simulink library "cstblocks"  (R2025b)
settings: Solver=ode45  StartTime=0.0  StopTime=10.0  RelTol=1e-3
values from neighbouring files (symbols this model uses):
  D = ltipack.lftdataFRD(IC,ltipack.LFTBlockWrapper(blk))    [ControlDesignBlock.m]    (also in DynamicBlock.m = pidstd(ltipack_ssdata(blk)); delayss.m = ltipack.ssdata(a0,b,c,[d0 q;s zeros(length(tau))],[],Ts))
  Ts = blk.Ts_    [DynamicBlock.m]    (also in delayss.m = varargin{1})
undefined symbols (not defined in the file or in its folder): AA, BB, CC, DD, Discrete, INFO, rss, set, Time, uDelay, V, xinit, yDelay
libraries: $bdroot x4, slpidlib x4, cstextras x4, sharedTrackingLibrary x3, ctrlSharedLib x1
(part 1 of 3)
settings Model: RequirementInfo=9  FPTRunName=Active  Creator=The MathWorks, Inc.  LastModifiedBy=The MathWorks, Inc.
settings SolverCC: AlgebraicLoopSolver=TrustRegion  MaxZcPerStep=1.0
settings DataIOCC: LimitDataPoints=on  SaveFormat=Array  SignalLoggingSaveFormat=ModelDataLogs  ReturnWorkspaceOutputs=off
settings OptimizationCC: BlockReduction=off  BooleanDataType=off  ExpressionDepthLimit=2147483647.0  LifeSpan=inf
settings DebuggingCC: SaveWithParameterizedLinksMsg=none  UnderspecifiedInitializationDetection=Classic  MergeDetectMultiDrivingBlocksExec=none  SignalResolutionControl=TryResolveAllWithWarning  FcnCallInpInsideContextMsg=warning  UnconnectedInputMsg=warning  UnconnectedOutputMsg=warning  UnconnectedLineMsg=warning  StateNameClashWarn=warning  SFUnexpectedBacktrackingDiag=warning  SFNoUnconditionalDefaultTransitionDiag=warning  SFExecutionAtInitializationDiag=none  ArithmeticOperatorsInVariantConditions=warning
settings HardwareCC: ProdBitPerPointer=32.0  ProdBitPerSizeT=32.0  ProdBitPerPtrDiffT=32.0  ProdLargestAtomicFloat=None  ProdIntDivRoundTo=Undefined  ProdEndianess=Unspecified  ProdWordSize=32.0  ProdHWDeviceType=32-bit Generic  TargetUnknown=on
settings ModelReferenceCC: EnableRefExpFcnMdlSchedulingChecks=on  PropagateSignalLabelsOutOfModel=off
settings SFSimCC: SimUseLocalCustomCode=off  CustomCodeUndefinedFunction=UseInterfaceOnly
settings RTWCC: RTWUseLocalCustomCode=off  GPUComputeCapability=3.5  DLArmComputeVersion=19.05  LargeConstantGeneration=WriteOnlyDNNConstantsToDataFiles
settings CodeAppCC: StateflowObjectComments=on
settings GRTTargetCC: TargetLangStandard=C89/C90 (ANSI)  CombineOutputUpdateFcns=off  GRTInterface=on
settings ConfigComp: CovMetricSettings=dw  CovSaveCumulativeToWorkspaceVar=on  CovSaveSingleToWorkspaceVar=on  CovExternalEMLEnable=off  CovSFcnEnable=off

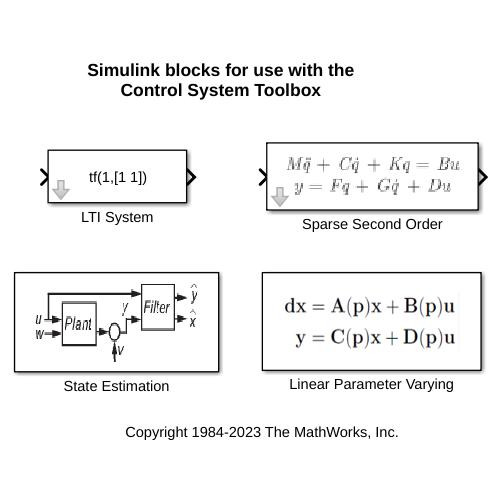
[thumbnail: Simulink's stored preview of the top-level diagram]
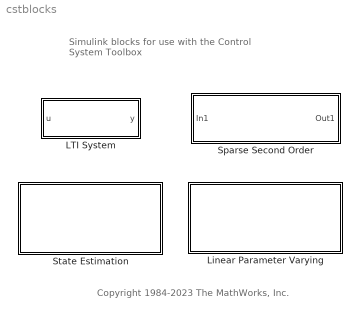
== system cstblocks ==
  note: Simulink blocks for use with the
      | Control System Toolbox
  note: Copyright 1984-2023 The MathWorks, Inc.
  LTI System : Subsystem  BlockChoice=CSS  mask(LTI Block){sys=tf(1,[1 1]), IC=[], PadeOrder=0}
      mask prompts: sys "Control:simulink:LTIMaskLabel1"; IC "Control:simulink:LTIMaskLabel2"; PadeOrder "Pade Order (for linearization)"
      mask help: Control:simulink:LTIMaskDescription
      mask init:
      | model = bdroot;
      | df = get_param(model,'dirty');
      | try
      |     [D,uDelay,yDelay,xinit,Ts,sysname] = controllib.internal.blocks.lti.ltimaskData(gcb,sys,IC);
      | catch ME
      |     sysname = '???';
      |     throwAsCaller(MSLException(get_param(gcb,'handle'),ME.identifier,ME.message))
      | end
      | controllib.internal.blocks.lti.ltimaskUpdate(gcb,D,xinit,Ts,PadeOrder)
      | try
      |     % Attempt to modify locked library -> error
      |     set_param(model,'dirty',df)
      | end
      mask Help: eval('helpview(''control'',''ltisystemblock'');')
      mask Callback sys: controllib.internal.blocks.lti.ltimaskCallback(gcb,'System')
      mask DialogControl sys Prompt: LTI system variable
      mask DialogControl IC Prompt: Initial states (state-space only)
      mask Display: disp(sysname)
  Linear Parameter Varying : Subsystem
      mask Display: image('lpv.png',[.1 .2 .8 .6])
  Sparse Second Order : Subsystem  mask(Sparse Second Order){M=1, C=0, K=1, B=1, F=1, G=0, D=0, q0=0, dq0=0}
      mask prompts: M "Control:simulink:SparseSecondOrder1"; C "Control:simulink:SparseSecondOrder2"; K "Control:simulink:SparseSecondOrder3"; q0 "Control:simulink:SparseSecondOrder4"; dq0 "Control:simulink:SparseSecondOrder5"
      mask help: Control:simulink:SSODescription
      mask init:
      | hCB = get_param(gcb,'handle');  % block handle
      | try
      |    sys = mechss(M,C,K,B,F,G,D);
      |    [AA,BB,CC,DD,EE] = sparssdata(sys);
      |    x0 = getx0(sys,q0,dq0);
      | catch ME
      |    throwAsCaller(MSLException(hCB, ME.identifier, ME.message));
      | end
      mask Help: eval('helpview(''control'',''ssoblock'');')
      mask DialogControl M Prompt: M (mass):
      mask DialogControl C Prompt: C (damping):
      mask DialogControl K Prompt: K (stiffness):
      mask DialogControl q0 Prompt: Initial position q(0):
      mask DialogControl dq0 Prompt: Initial velocity q'(0):
  State Estimation : Subsystem
      mask Display: image('kalman.png',[0.1 0.1 0.8 0.8])

== system cstblocks/LTI System ==
  u : Inport  PortDimensions=1  SampleTime=Ts
  Input Delay : $bdroot/Linear Parameter Varying/Varying Delay  Td=uDelay  TdMax=max(uDelay)  TdMin=0  TdFixed=1  u0=0  bufsize=1024  FixedBuffer=off  PadeOrder=0
  Internal : StateSpace  A=D.a  B=D.b  C=D.c  D=D.d  InitialCondition=xinit
  Output Delay : $bdroot/Linear Parameter Varying/Varying Delay  Td=yDelay  TdMax=max(yDelay)  TdMin=0  TdFixed=1  u0=0  bufsize=1024  FixedBuffer=off  PadeOrder=0
  y : Outport  InitialOutput=0  VectorParamsAs1DForOutWhenUnconnected=off
  wires:
  u/1 -> Input Delay/1
  Output Delay/1 -> y/1
  Input Delay/1 -> Internal/1
  Internal/1 -> Output Delay/1
